simulink model "SensorTryout"  (R2022a)
settings: Solver=ode15s  StartTime=0.0  StopTime=10.0  RelTol=1e-3
values from neighbouring files (symbols this model uses):
  C = eye(6)    [Gyro.m]
undefined symbols (not defined in the file or in its folder): Newton, Raphson
libraries: sim3dphyssensorlib x3, sim3dprobsensorlib x3, uavalgslib x1, trackingutilitieslib x1, sim3dlib x1, uavsim3dlib x1
settings Model: Creator=korne  LastModifiedBy=korne

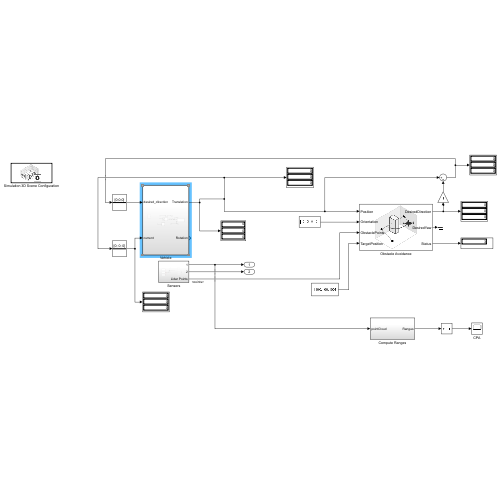
[thumbnail: Simulink's stored preview of the top-level diagram]
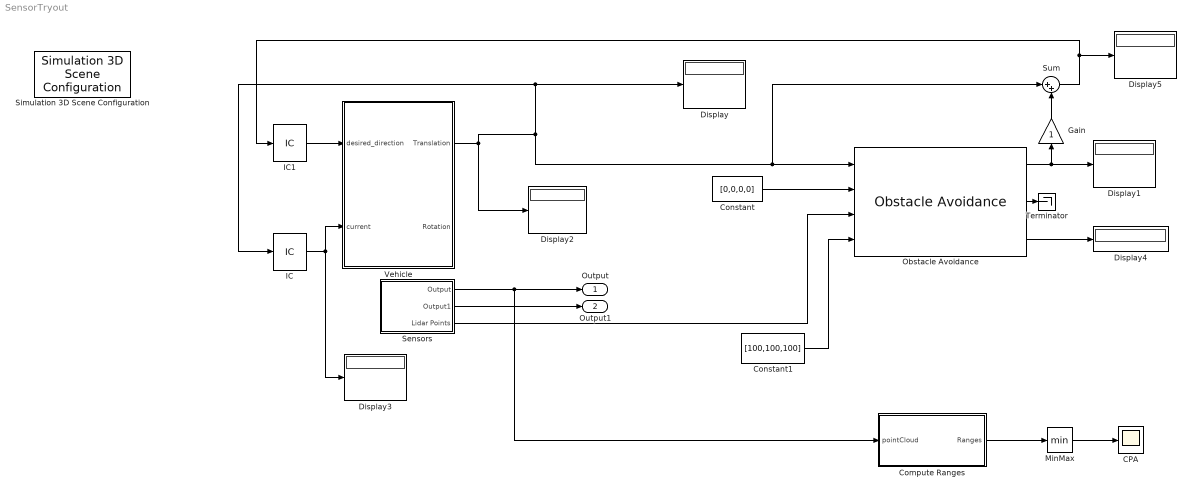
== system SensorTryout ==
  CPA : Scope
  Compute Ranges : Subsystem
  Constant : Constant  Value=[0,0,0,0]
  Constant1 : Constant  Value=[100,100,100]
  Display{,1..5} (6 alike) : Display
  Gain : Gain
  IC : InitialCondition  Value=[0; 0; 0]
  IC1 : InitialCondition  Value=[0;0;0]
  MinMax : MinMax
  Obstacle Avoidance : uavalgslib/Obstacle Avoidance  DistanceLimits=[ 0.2, 10 ]  HorizontalSensorFOV=[ -180, 180 ]  VerticalSensorFOV=[ -30, 30 ]  SensorLocation=[0, 0, -.1]  SensorOrientation=[ 0, -pi/2, 0 ]  VehicleRadius=1  SafetyDistance=1  SimulateUsing=Code generation  HistRes=5  WindowSize=1  HistogramThreshold=1  MaxAge=0  TargetDirectionWeight=5  CurrentDirectionWeight=2  PreviousDirectionWeight=2
      settings: SourceProductBaseCode=UV
  Sensors : Subsystem
  Simulation 3D Scene Configuration : sim3dlib/Simulation 3D Scene Configuration  Priority=0  ProjectFormat=Default Scenes  SceneDesc=US city block  ProjectName=C:\TuDelft\toolbox\shared\sim3d_projects\automotive_project\UE4\WindowsNoEditor\VehicleSimulation.exe  ScenePath=/Game/Maps/USCityBlock  vehTagList={'Scene Origin';'SimulinkVehicle1'}  vehTag=SimulinkVehicle1  OpVisEn=off  Ts=1/15  EnableWindow=on  EnableRemoteAccess=off  EnableWeather=on  SunAltitude=40.0  SunAzimuth=90  clouds=10  wind=1  fog=0  rain=20.0  sensorTag=MainCamera1  sensorId=1  sensorName=MainCamera1  mountLoc=Origin  offsetFlag=off  tmountOffset=[0, 0, 0]  rmountOffset=[0, 0, 0]  HorizontalResolution=1280  VerticalResolution=720  HorizontalFOV=60  mountPoint=[0 0 0]  mountOrientation=[0 0 0]  aMode=4  ID=1
      settings: SourceProductBaseCode=VE,AE,DR,UV,VE
  Sum : Sum  Inputs=|++
  Terminator : Terminator
  Vehicle : Subsystem
  Output : Outport
  Output1 : Outport  Port=2
  wires:
  Sensors/1(Output) -> Compute Ranges/1(pointCloud), Output/1
  Sensors/2(Output1) -> Output1/1
  Constant/1 -> Obstacle Avoidance/2
  Constant1/1 -> Obstacle Avoidance/4
  Obstacle Avoidance/1 -> Display1/1, Gain/1
  Obstacle Avoidance/2 -> Terminator/1
  Obstacle Avoidance/3 -> Display4/1
  IC1/1 -> Vehicle/1(desired_direction)
  Vehicle/1(Translation) -> IC/1, Display/1, Sum/1, Obstacle Avoidance/1, Display2/1
  IC/1 -> Vehicle/2(current), Display3/1
  Gain/1 -> Sum/2
  Sum/1 -> Display5/1, IC1/1
  Compute Ranges/1(Ranges) -> MinMax/1
  MinMax/1 -> CPA/1
  Sensors/3(Lidar Points) -> Obstacle Avoidance/3

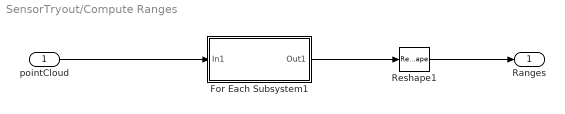
== system SensorTryout/Compute Ranges ==
  pointCloud : Inport
  For Each Subsystem1 : Subsystem  TreatAsAtomicUnit=on
  Reshape1 : Reshape  OutputDimensions=1083
  Ranges : Outport
  wires:
  For Each Subsystem1/1(Out1) -> Reshape1/1
  pointCloud/1 -> For Each Subsystem1/1(In1)
  Reshape1/1 -> Ranges/1

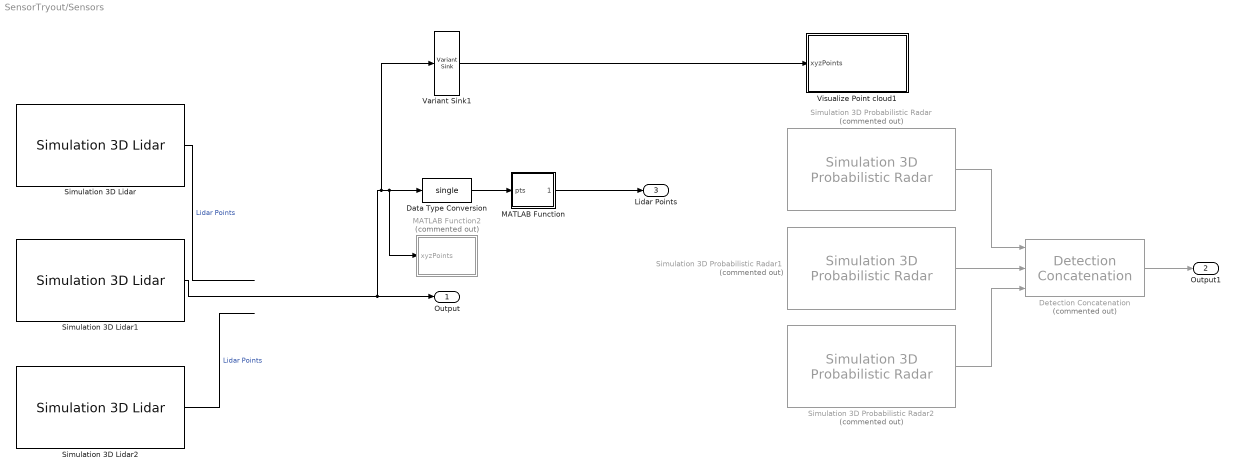
== system SensorTryout/Sensors ==
  Data Type Conversion : DataTypeConversion  OutDataTypeStr=single  SaturateOnIntegerOverflow=off  RndMeth=Floor
  Detection Concatenation : trackingutilitieslib/Detection Concatenation  Commented=on  NumInputs=3  BusNameSource=Auto  BusName=BusDetectionConcatenation  SimulateUsing=Interpreted execution
      settings: SourceProductBaseCode=TF,AE,DR,RA,UV,VE
  MATLAB Function : MATLAB Function  TreatAsAtomicUnit=on
  MATLAB Function2 : MATLAB Function  Commented=on  TreatAsAtomicUnit=on
  Simulation 3D Lidar : sim3dphyssensorlib/Simulation 3D Lidar  Priority=1  sensorTag=Sim3dSensor1  sensorId=1  sensorName=Sim3dSensor1  vehTagList={'Scene Origin';'SimulinkVehicle1'}  vehTag=SimulinkVehicle1  mountLoc=Origin  offsetFlag=on  tmountOffset=[0, 0, 1]  rmountOffset=[0, pi/2, 0]  DetectionRange=100  RangeResolution=0.002  VerticalFOV=90  VerticalResolution=1.25  HorizontalFOV=360  HorizontalResolution=0.16  DistanceOutportEnabled=off  ReflectivityOutportEnabled=off  TransformOutportEnabled=off  SampleTime=-1  mountPoint=[0 0 1]  mountOrientation=[0 -1.5707963267949 0]  aMode=4  ID=1
      settings: SourceProductBaseCode=VE,AE,DR,UV,VE
  Simulation 3D Lidar1 : sim3dphyssensorlib/Simulation 3D Lidar  Priority=1  sensorTag=Sim3dSensor6  sensorId=6  sensorName=Sim3dSensor6  vehTagList={'Scene Origin';'SimulinkVehicle1'}  vehTag=SimulinkVehicle1  mountLoc=Origin  offsetFlag=on  tmountOffset=[0, 0, -.1]  rmountOffset=[0, -pi/2, 0]  DetectionRange=100  RangeResolution=0.002  VerticalFOV=90  VerticalResolution=1.25  HorizontalFOV=360  HorizontalResolution=0.16  DistanceOutportEnabled=off  ReflectivityOutportEnabled=off  TransformOutportEnabled=off  SampleTime=-1  mountPoint=[0 0 -0.1]  mountOrientation=[0 1.5707963267949 0]  aMode=4  ID=6
      settings: SourceProductBaseCode=VE,AE,DR,UV,VE
  Simulation 3D Lidar2 : sim3dphyssensorlib/Simulation 3D Lidar  Priority=1  sensorTag=Sim3dSensor7  sensorId=7  sensorName=Sim3dSensor7  vehTagList={'Scene Origin';'SimulinkVehicle1'}  vehTag=SimulinkVehicle1  mountLoc=Origin  offsetFlag=on  tmountOffset=[1, 0, 0]  rmountOffset=[0,0, 0]  DetectionRange=100  RangeResolution=0.002  VerticalFOV=90  VerticalResolution=1.25  HorizontalFOV=360  HorizontalResolution=0.16  DistanceOutportEnabled=off  ReflectivityOutportEnabled=off  TransformOutportEnabled=off  SampleTime=-1  mountPoint=[1 0 0]  mountOrientation=[0 0 0]  aMode=4  ID=7
      settings: SourceProductBaseCode=VE,AE,DR,UV,VE
  Simulation 3D Probabilistic Radar : sim3dprobsensorlib/Simulation 3D Probabilistic Radar  Priority=1  Commented=on  sensorTag=Sim3dSensor2  sensorId=2  sensorName=Sim3dSensor2  vehTagList={'Scene Origin';'SimulinkVehicle1'}  vehTag=SimulinkVehicle1  mountLoc=Origin  offsetFlag=on  tmountOffset=[0, 0, 0]  rmountOffset=[0, 0, 0]  AzimuthResolution=4  ElevationResolution=10  RangeResolution=2.5  RangeRateResolution=0.5  AzimuthBiasFraction=0.1  ElevationBiasFraction=0.1  RangeBiasFraction=0.05  RangeRateBiasFraction=0.05  FieldOfView=[ 20, 5 ]  DetectionRange=[ 1, 150 ]  RangeRateLimits=[ -100, 100 ]  DetectionProbability=0.9  FalseAlarmRate=1e-6  ReferenceRange=100  ReferenceRCS=0  HasElevation=on  HasRangeRate=on  HasNoise=on  HasFalseAlarms=on  InitialSeedSource=Repeatable  InitialSeed=0  MaxNumDetections=50  DetectionCoordinates=Ego Cartesian  SpecifyOutputBusName=off  BusName=BusSimulation3DRadarTruthSensor  SampleTime=-1  mountPoint=[0 0 0]  mountOrientation=[0 0 0]  aMode=3  ID=2
      settings: SourceProductBaseCode=VE,AE,DR,UV,VE
  Simulation 3D Probabilistic Radar1 : sim3dprobsensorlib/Simulation 3D Probabilistic Radar  Priority=1  Commented=on  sensorTag=Sim3dSensor4  sensorId=4  sensorName=Sim3dSensor4  vehTagList={'Scene Origin';'SimulinkVehicle1'}  vehTag=SimulinkVehicle1  mountLoc=Origin  offsetFlag=on  tmountOffset=[0, 0, 0]  rmountOffset=[0, 0, 90]  AzimuthResolution=4  ElevationResolution=10  RangeResolution=2.5  RangeRateResolution=0.5  AzimuthBiasFraction=0.1  ElevationBiasFraction=0.1  RangeBiasFraction=0.05  RangeRateBiasFraction=0.05  FieldOfView=[ 20, 5 ]  DetectionRange=[ 1, 150 ]  RangeRateLimits=[ -100, 100 ]  DetectionProbability=0.9  FalseAlarmRate=1e-6  ReferenceRange=100  ReferenceRCS=0  HasElevation=on  HasRangeRate=on  HasNoise=on  HasFalseAlarms=on  InitialSeedSource=Repeatable  InitialSeed=0  MaxNumDetections=50  DetectionCoordinates=Ego Cartesian  SpecifyOutputBusName=off  BusName=BusSimulation3DRadarTruthSensor  SampleTime=-1  mountPoint=[0 0 0]  mountOrientation=[0 0 -90]  aMode=3  ID=4
      settings: SourceProductBaseCode=VE,AE,DR,UV,VE
  Simulation 3D Probabilistic Radar2 : sim3dprobsensorlib/Simulation 3D Probabilistic Radar  Priority=1  Commented=on  sensorTag=Sim3dSensor5  sensorId=5  sensorName=Sim3dSensor5  vehTagList={'Scene Origin';'SimulinkVehicle1'}  vehTag=SimulinkVehicle1  mountLoc=Origin  offsetFlag=on  tmountOffset=[0, 0, 0]  rmountOffset=[0, 0, 180]  AzimuthResolution=4  ElevationResolution=10  RangeResolution=2.5  RangeRateResolution=0.5  AzimuthBiasFraction=0.1  ElevationBiasFraction=0.1  RangeBiasFraction=0.05  RangeRateBiasFraction=0.05  FieldOfView=[ 20, 5 ]  DetectionRange=[ 1, 150 ]  RangeRateLimits=[ -100, 100 ]  DetectionProbability=0.9  FalseAlarmRate=1e-6  ReferenceRange=100  ReferenceRCS=0  HasElevation=on  HasRangeRate=on  HasNoise=on  HasFalseAlarms=on  InitialSeedSource=Repeatable  InitialSeed=0  MaxNumDetections=50  DetectionCoordinates=Ego Cartesian  SpecifyOutputBusName=off  BusName=BusSimulation3DRadarTruthSensor  SampleTime=-1  mountPoint=[0 0 0]  mountOrientation=[0 0 -180]  aMode=3  ID=5
      settings: SourceProductBaseCode=VE,AE,DR,UV,VE
  Variant Sink1 : VariantSink
      settings: AllowZeroVariantControls=on
  Visualize Point cloud1 : MATLAB Function  StopFcn=|  TreatAsAtomicUnit=on
      | playerFigure = findall(groot,'type','figure','name','Point Cloud Player');
      | 
      | if ~isempty(playerFigure)
      |     playerFigure = playerFigure(end);
      |     if isvalid(playerFigure)
      |         close(playerFigure);
      |     end
      | end
  Output : Outport
  Output1 : Outport  Port=2
  Lidar Points : Outport  Port=3
  wires:
  Simulation 3D Probabilistic Radar/1 -> Detection Concatenation/1
  Detection Concatenation/1 -> Output1/1
  Simulation 3D Probabilistic Radar1/1 -> Detection Concatenation/2
  Simulation 3D Probabilistic Radar2/1 -> Detection Concatenation/3
  Data Type Conversion/1 -> MATLAB Function/1(pts)
  MATLAB Function/1(points) -> Lidar Points/1
  Simulation 3D Lidar/1 -> ?  "Lidar Points"
  Simulation 3D Lidar2/1 -> ?  "Lidar Points"
  Variant Sink1/1 -> Visualize Point cloud1/1(xyzPoints)
  Simulation 3D Lidar1/1 -> Variant Sink1/1, Data Type Conversion/1, MATLAB Function2/1(xyzPoints), Output/1

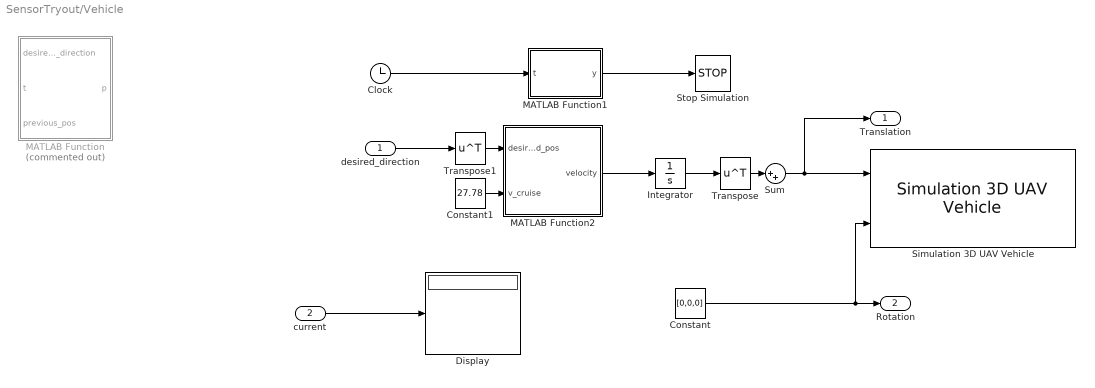
== system SensorTryout/Vehicle ==
  desired_direction : Inport
  current : Inport  Port=2
  Clock : Clock
  Constant : Constant  Value=[0,0,0]
  Constant1 : Constant  Value=27.78
  Display : Display
  Integrator : Integrator
  MATLAB Function : MATLAB Function  Commented=on  TreatAsAtomicUnit=on
  MATLAB Function1 : MATLAB Function  TreatAsAtomicUnit=on
  MATLAB Function2 : MATLAB Function  TreatAsAtomicUnit=on
  Simulation 3D UAV Vehicle : uavsim3dlib/Simulation 3D UAV Vehicle  Priority=-1  Mesh=Quadrotor  MeshPath=/MathWorksUAVContent/UAVs/HexaRotorUAV/HexaRotor.HexaRotor  Color=Orange  ActorName=SimulinkVehicle1  InitialTranslation=[0,0,0]  InitialRotation=[0 0 0]  SampleTime=-1  ActorType=SimulinkVehicle  ID=1  aMode=4  ActorTag=SimulinkVehicle1
      settings: SourceProductBaseCode=UV
  Stop Simulation : Stop
  Sum : Sum  Inputs=|++
  Transpose : Math  Operator=transpose
  Transpose1 : Math  Operator=transpose
  Translation : Outport
  Rotation : Outport  Port=2
  wires:
  MATLAB Function1/1(y) -> Stop Simulation/1
  Clock/1 -> MATLAB Function1/1(t)
  Constant/1 -> Simulation 3D UAV Vehicle/2, Rotation/1
  desired_direction/1 -> Transpose1/1
  current/1 -> Display/1
  MATLAB Function2/1(velocity) -> Integrator/1
  Sum/1 -> Simulation 3D UAV Vehicle/1, Translation/1
  Transpose/1 -> Sum/1
  Constant1/1 -> MATLAB Function2/2(v_cruise)
  Integrator/1 -> Transpose/1
  Transpose1/1 -> MATLAB Function2/1(desired_pos)

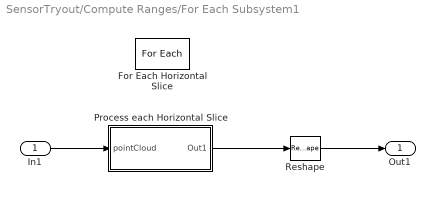
== system SensorTryout/Compute Ranges/For Each Subsystem1 ==
  In1 : Inport  Partition=on  PartitionDimension=1  PartitionWidth=1  PartitionOffset=0
  For Each Horizontal Slice : ForEach  DisableCoverage=on
  Process each Horizontal Slice : Subsystem  TreatAsAtomicUnit=on
  Reshape : Reshape
  Out1 : Outport  ConcatenationDimension=1
  wires:
  In1/1 -> Process each Horizontal Slice/1(pointCloud)
  Process each Horizontal Slice/1(Out1) -> Reshape/1
  Reshape/1 -> Out1/1

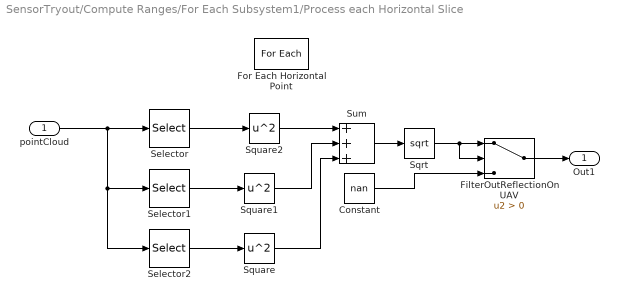
== system SensorTryout/Compute Ranges/For Each Subsystem1/Process each Horizontal Slice ==
  pointCloud : Inport  Partition=on  PartitionDimension=2  PartitionWidth=1  PartitionOffset=0
  Constant : Constant  Value=nan
  FilterOutReflectionOnUAV : Switch  Criteria=u2 > Threshold  SaturateOnIntegerOverflow=off  InputSameDT=off
  For Each Horizontal Point : ForEach  DisableCoverage=on
  Selector : Selector  NumberOfDimensions=3  InputPortWidth=3  IndexOptions=Index vector (dialog),Index vector (dialog),Index vector (dialog)  Indices=1,1,1  OutputSizes=1,1,1
  Selector1 : Selector  NumberOfDimensions=3  InputPortWidth=3  IndexOptions=Index vector (dialog),Index vector (dialog),Index vector (dialog)  Indices=1,1,2  OutputSizes=1,1,1
  Selector2 : Selector  NumberOfDimensions=3  InputPortWidth=3  IndexOptions=Index vector (dialog),Index vector (dialog),Index vector (dialog)  Indices=1,1,3  OutputSizes=1,1,1
  Sqrt : Sqrt  OutputSignalType=real  OutDataTypeStr=single  IntermediateResultsDataTypeStr=single  AlgorithmType=Newton-Raphson
  Square : Math  Operator=square
  Square1 : Math  Operator=square
  Square2 : Math  Operator=square
  Sum : Sum  Inputs=+++
  Out1 : Outport  ConcatenationDimension=1
  wires:
  pointCloud/1 -> Selector2/1, Selector1/1, Selector/1
  Selector/1 -> Square2/1
  Selector1/1 -> Square1/1
  Square2/1 -> Sum/1
  Square1/1 -> Sum/2
  Sum/1 -> Sqrt/1
  Sqrt/1 -> FilterOutReflectionOnUAV/1, FilterOutReflectionOnUAV/2
  Selector2/1 -> Square/1
  Square/1 -> Sum/3
  FilterOutReflectionOnUAV/1 -> Out1/1
  Constant/1 -> FilterOutReflectionOnUAV/3

== matlab function SensorTryout/Vehicle/MATLAB Function1 ==
  data: t input; y output
function y = fcn(t)
if t < 11
    y = 0;
else
    y = t;
end

== matlab function SensorTryout/Vehicle/MATLAB Function ==
  data: desired_direction input; t input; p output; previous_pos input
function p = fcn(desired_direction, t, previous_pos)
v_max = 100/3.6;
gamma = atan(desired_direction(3)/sqrt(desired_direction(1)^2+desired_direction(2)^2)); %angle between z and xy plane
beta  = atan(desired_direction(2)/desired_direction(1));

dt = 0.1;
x = dt*cos(beta)*v_max + previous_pos(1);
y = dt*sin(beta)*v_max + previous_pos(2);
z = dt*sin(gamma)*v_max + previous_pos(3);

p = [x,y,z];

== matlab function SensorTryout/Sensors/MATLAB Function2 ==
  data: xyzPoints input
function VisualizePointCloud(xyzPoints)
%VisualizePointCloud Display point cloud

coder.extrinsic('isOpen', 'pcplayer')

persistent player;

if isempty(player)
    % Configure axes limits
    xlimits = [-90 90];
    ylimits = [-90 90];
    zlimits = [ -5 40];
    
    % Create a streaming Lidar viewer
    player = pcplayer(xlimits, ylimits, zlimits);
end

if ~isempty(player) && isOpen(player)
    view(player, xyzPoints);
end

== matlab function SensorTryout/Sensors/MATLAB Function ==
  data: pts input; points output
function points = lidarToPoints(pts)

xLidar = reshape(pts(:,:,1),[],1);
yLidar = reshape(pts(:,:,2),[],1);
zLidar = reshape(pts(:,:,3),[],1);
    
points = [xLidar,yLidar,zLidar];

== matlab function SensorTryout/Vehicle/MATLAB Function2 ==
  data: desired_pos input; velocity output; v_cruise input
function velocity = v_vector(desired_pos, v_cruise)
if desired_pos == [0,0,0]
    velocity = [0,0,0];
    return
end
desired_pos_norm = desired_pos/norm(desired_pos);

velocity = desired_pos_norm*v_cruise;

== matlab function SensorTryout/Sensors/Visualize Point cloud1 ==
  data: xyzPoints input
function VisualizePointCloud(xyzPoints)
%VisualizePointCloud Display point cloud

coder.extrinsic('isOpen', 'pcplayer')

persistent player;

if isempty(player)
    % Configure axes limits
    xlimits = [-90 90];
    ylimits = [-90 90];
    zlimits = [ -50 50];
    
    % Create a streaming Lidar viewer
    player = pcplayer(xlimits, ylimits, zlimits);
end

if ~isempty(player) && isOpen(player)
    view(player, xyzPoints);
end
